simulink model "Project2"  (R2021a)
settings: Solver=VariableStepAuto  StartTime=0.0  StopTime=16  RelTol=1e-3
libraries: hdlBasic x209, dspsrcs4 x2, xbsIndex_r4 x1, hlsBasic x1
(part 1 of 2)
settings Model: Creator=caval  LastModifiedBy=user

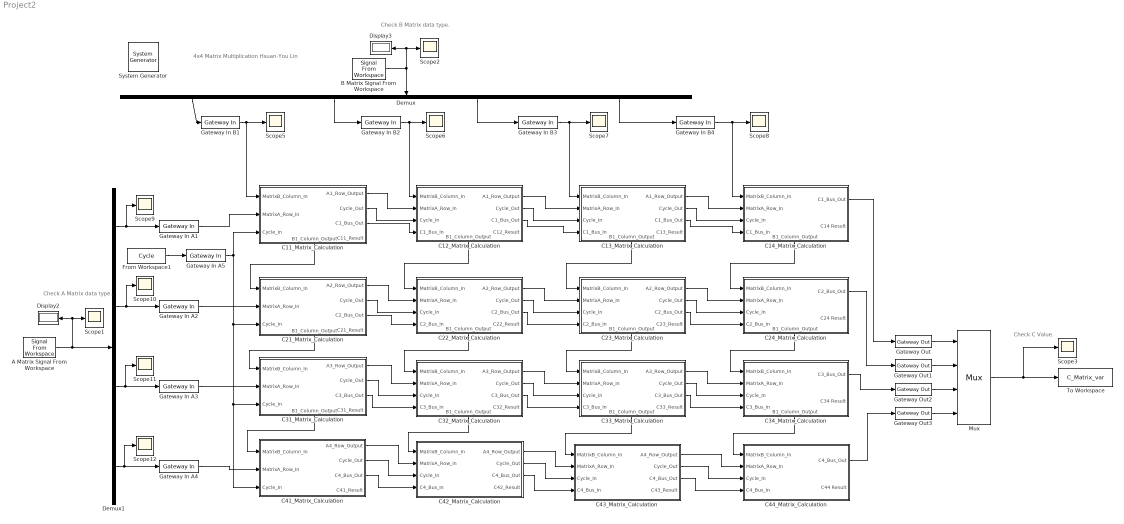
== system Project2 ==
  note: 4x4 Matrix Multiplication
      | Hsuan-You Lin
  note: Check A Matrix data type.
  note: Check B Matrix data type.
  note: Check C Value.
  " System Generator" : xbsIndex_r4/ System Generator  Tag=genX  xilinxfamily=zynq  part=xc7z020  speed=-1  package=clg484  synthesis_tool=Vivado  clock_wrapper=Clock Enables  directory=./netlist  proj_type=Vivado  Synth_file=Vivado Synthesis Defaults  Impl_file=Vivado Implementation Defaults  testbench=off  simulink_period=1  sysclk_period=7  dcm_input_clock_period=10  incr_netlist=off  trim_vbits=Everywhere in SubSystem  dbl_ovrd=According to Block Masks  core_generation=According to Block Masks  run_coregen=off  deprecated_control=off  eval_field=0  block_type=sysgen
  A Matrix Signal From Workspace : dspsrcs4/Signal From Workspace  X=A_Input  Ts=1  nsamps=1  OutputAfterFinalValue=Setting to zero  ignoreOrWarnInputAndFrameLengths=off  OutputFrames=off
  B Matrix Signal From Workspace : dspsrcs4/Signal From Workspace  X=B_Input  Ts=1  nsamps=1  OutputAfterFinalValue=Setting to zero  ignoreOrWarnInputAndFrameLengths=off  OutputFrames=off
  C11_Matrix_Calculation : Subsystem
      settings: PortSchema="{\"entries\":[{\"content\":{\"sides\":[{\"content\":{\"connectorIds\":[\"In1\",\"In2\",\"In3\"]},\"type\":\"ConnectorPlacement.EquallySpacedRectSide\",\"uuid\":\"74ab6ecd-cc08-4ee4-ac19-9cc8be9c6472\"},{\"content\":{\"connectorIds\":[\"Out1\",\"Out2\",\"Out3\",\"Out4\"],\"side\":\"RIGHT\"},\"type\":\"ConnectorPlacement.EquallySpacedRectSide\",\"uuid\":\"1cd07b35-dcc9-4612-a415-f960f8d5f61b\"},{\"content\":{\"connectorIds\":[],\"side\":\"TOP\"},\"type\":\"ConnectorPlacement.EquallySpacedRectSide\",\"uuid\":\"476a3fdc-a239-49e7-9d04-c8df306fd8f0\"},{\"content\":{\"connectorIds\":[\"Out5\"],\"side\":\"BOTTOM\"},\"type\":\"ConnectorPlacement.EquallySpacedRectSide\",\"uuid\":\"4811719c-b9ad-4f94-b919-bfccafa53e00\"}]},\"type\":\"ConnectorPlacement.EquallySpacedConnector\",\"uuid\":\"06e904f9-bca4-4dcb-a7b8-01e13ea2fc40\"}],\"packageUris\":[\"http://schema.mathworks.com/mf0/Connector/R2020b\"],\"version\":\"1.0\"}"
  C12_Matrix_Calculation : Subsystem
      settings: PortSchema="{\"entries\":[{\"content\":{\"sides\":[{\"content\":{\"connectorIds\":[\"In1\",\"In2\",\"In3\",\"In4\"]},\"type\":\"ConnectorPlacement.EquallySpacedRectSide\",\"uuid\":\"74ab6ecd-cc08-4ee4-ac19-9cc8be9c6472\"},{\"content\":{\"connectorIds\":[\"Out1\",\"Out2\",\"Out3\",\"Out4\"],\"side\":\"RIGHT\"},\"type\":\"ConnectorPlacement.EquallySpacedRectSide\",\"uuid\":\"1cd07b35-dcc9-4612-a415-f960f8d5f61b\"},{\"content\":{\"connectorIds\":[],\"side\":\"TOP\"},\"type\":\"ConnectorPlacement.EquallySpacedRectSide\",\"uuid\":\"476a3fdc-a239-49e7-9d04-c8df306fd8f0\"},{\"content\":{\"connectorIds\":[\"Out5\"],\"side\":\"BOTTOM\"},\"type\":\"ConnectorPlacement.EquallySpacedRectSide\",\"uuid\":\"4811719c-b9ad-4f94-b919-bfccafa53e00\"}]},\"type\":\"ConnectorPlacement.EquallySpacedConnector\",\"uuid\":\"06e904f9-bca4-4dcb-a7b8-01e13ea2fc40\"}],\"packageUris\":[\"http://schema.mathworks.com/mf0/Connector/R2020b\"],\"version\":\"1.0\"}"
  C13_Matrix_Calculation : Subsystem
      settings: PortSchema="{\"entries\":[{\"content\":{\"sides\":[{\"content\":{\"connectorIds\":[\"In1\",\"In2\",\"In3\",\"In4\"]},\"type\":\"ConnectorPlacement.EquallySpacedRectSide\",\"uuid\":\"74ab6ecd-cc08-4ee4-ac19-9cc8be9c6472\"},{\"content\":{\"connectorIds\":[\"Out1\",\"Out2\",\"Out3\",\"Out4\"],\"side\":\"RIGHT\"},\"type\":\"ConnectorPlacement.EquallySpacedRectSide\",\"uuid\":\"1cd07b35-dcc9-4612-a415-f960f8d5f61b\"},{\"content\":{\"connectorIds\":[],\"side\":\"TOP\"},\"type\":\"ConnectorPlacement.EquallySpacedRectSide\",\"uuid\":\"476a3fdc-a239-49e7-9d04-c8df306fd8f0\"},{\"content\":{\"connectorIds\":[\"Out5\"],\"side\":\"BOTTOM\"},\"type\":\"ConnectorPlacement.EquallySpacedRectSide\",\"uuid\":\"4811719c-b9ad-4f94-b919-bfccafa53e00\"}]},\"type\":\"ConnectorPlacement.EquallySpacedConnector\",\"uuid\":\"06e904f9-bca4-4dcb-a7b8-01e13ea2fc40\"}],\"packageUris\":[\"http://schema.mathworks.com/mf0/Connector/R2020b\"],\"version\":\"1.0\"}"
  C14_Matrix_Calculation : Subsystem
      settings: PortSchema="{\"entries\":[{\"content\":{\"sides\":[{\"content\":{\"connectorIds\":[\"In1\",\"In2\",\"In3\",\"In4\"]},\"type\":\"ConnectorPlacement.EquallySpacedRectSide\",\"uuid\":\"74ab6ecd-cc08-4ee4-ac19-9cc8be9c6472\"},{\"content\":{\"connectorIds\":[\"Out1\",\"Out2\"],\"side\":\"RIGHT\"},\"type\":\"ConnectorPlacement.EquallySpacedRectSide\",\"uuid\":\"1cd07b35-dcc9-4612-a415-f960f8d5f61b\"},{\"content\":{\"connectorIds\":[],\"side\":\"TOP\"},\"type\":\"ConnectorPlacement.EquallySpacedRectSide\",\"uuid\":\"476a3fdc-a239-49e7-9d04-c8df306fd8f0\"},{\"content\":{\"connectorIds\":[\"Out3\"],\"side\":\"BOTTOM\"},\"type\":\"ConnectorPlacement.EquallySpacedRectSide\",\"uuid\":\"4811719c-b9ad-4f94-b919-bfccafa53e00\"}]},\"type\":\"ConnectorPlacement.EquallySpacedConnector\",\"uuid\":\"06e904f9-bca4-4dcb-a7b8-01e13ea2fc40\"}],\"packageUris\":[\"http://schema.mathworks.com/mf0/Connector/R2020b\"],\"version\":\"1.0\"}"
  C21_Matrix_Calculation : Subsystem
      settings: PortSchema="{\"entries\":[{\"content\":{\"sides\":[{\"content\":{\"connectorIds\":[\"In1\",\"In2\",\"In3\"]},\"type\":\"ConnectorPlacement.EquallySpacedRectSide\",\"uuid\":\"74ab6ecd-cc08-4ee4-ac19-9cc8be9c6472\"},{\"content\":{\"connectorIds\":[\"Out1\",\"Out2\",\"Out3\",\"Out4\"],\"side\":\"RIGHT\"},\"type\":\"ConnectorPlacement.EquallySpacedRectSide\",\"uuid\":\"1cd07b35-dcc9-4612-a415-f960f8d5f61b\"},{\"content\":{\"connectorIds\":[],\"side\":\"TOP\"},\"type\":\"ConnectorPlacement.EquallySpacedRectSide\",\"uuid\":\"476a3fdc-a239-49e7-9d04-c8df306fd8f0\"},{\"content\":{\"connectorIds\":[\"Out5\"],\"side\":\"BOTTOM\"},\"type\":\"ConnectorPlacement.EquallySpacedRectSide\",\"uuid\":\"4811719c-b9ad-4f94-b919-bfccafa53e00\"}]},\"type\":\"ConnectorPlacement.EquallySpacedConnector\",\"uuid\":\"06e904f9-bca4-4dcb-a7b8-01e13ea2fc40\"}],\"packageUris\":[\"http://schema.mathworks.com/mf0/Connector/R2020b\"],\"version\":\"1.0\"}"
  C22_Matrix_Calculation : Subsystem
      settings: PortSchema="{\"entries\":[{\"content\":{\"sides\":[{\"content\":{\"connectorIds\":[\"In1\",\"In2\",\"In3\",\"In4\"]},\"type\":\"ConnectorPlacement.EquallySpacedRectSide\",\"uuid\":\"74ab6ecd-cc08-4ee4-ac19-9cc8be9c6472\"},{\"content\":{\"connectorIds\":[\"Out1\",\"Out2\",\"Out3\",\"Out4\"],\"side\":\"RIGHT\"},\"type\":\"ConnectorPlacement.EquallySpacedRectSide\",\"uuid\":\"1cd07b35-dcc9-4612-a415-f960f8d5f61b\"},{\"content\":{\"connectorIds\":[],\"side\":\"TOP\"},\"type\":\"ConnectorPlacement.EquallySpacedRectSide\",\"uuid\":\"476a3fdc-a239-49e7-9d04-c8df306fd8f0\"},{\"content\":{\"connectorIds\":[\"Out5\"],\"side\":\"BOTTOM\"},\"type\":\"ConnectorPlacement.EquallySpacedRectSide\",\"uuid\":\"4811719c-b9ad-4f94-b919-bfccafa53e00\"}]},\"type\":\"ConnectorPlacement.EquallySpacedConnector\",\"uuid\":\"06e904f9-bca4-4dcb-a7b8-01e13ea2fc40\"}],\"packageUris\":[\"http://schema.mathworks.com/mf0/Connector/R2020b\"],\"version\":\"1.0\"}"
  C23_Matrix_Calculation : Subsystem
      settings: PortSchema="{\"entries\":[{\"content\":{\"sides\":[{\"content\":{\"connectorIds\":[\"In1\",\"In2\",\"In3\",\"In4\"]},\"type\":\"ConnectorPlacement.EquallySpacedRectSide\",\"uuid\":\"74ab6ecd-cc08-4ee4-ac19-9cc8be9c6472\"},{\"content\":{\"connectorIds\":[\"Out1\",\"Out2\",\"Out3\",\"Out4\"],\"side\":\"RIGHT\"},\"type\":\"ConnectorPlacement.EquallySpacedRectSide\",\"uuid\":\"1cd07b35-dcc9-4612-a415-f960f8d5f61b\"},{\"content\":{\"connectorIds\":[],\"side\":\"TOP\"},\"type\":\"ConnectorPlacement.EquallySpacedRectSide\",\"uuid\":\"476a3fdc-a239-49e7-9d04-c8df306fd8f0\"},{\"content\":{\"connectorIds\":[\"Out5\"],\"side\":\"BOTTOM\"},\"type\":\"ConnectorPlacement.EquallySpacedRectSide\",\"uuid\":\"4811719c-b9ad-4f94-b919-bfccafa53e00\"}]},\"type\":\"ConnectorPlacement.EquallySpacedConnector\",\"uuid\":\"06e904f9-bca4-4dcb-a7b8-01e13ea2fc40\"}],\"packageUris\":[\"http://schema.mathworks.com/mf0/Connector/R2020b\"],\"version\":\"1.0\"}"
  C24_Matrix_Calculation : Subsystem
      settings: PortSchema="{\"entries\":[{\"content\":{\"sides\":[{\"content\":{\"connectorIds\":[\"In1\",\"In2\",\"In3\",\"In4\"]},\"type\":\"ConnectorPlacement.EquallySpacedRectSide\",\"uuid\":\"74ab6ecd-cc08-4ee4-ac19-9cc8be9c6472\"},{\"content\":{\"connectorIds\":[\"Out1\",\"Out2\"],\"side\":\"RIGHT\"},\"type\":\"ConnectorPlacement.EquallySpacedRectSide\",\"uuid\":\"1cd07b35-dcc9-4612-a415-f960f8d5f61b\"},{\"content\":{\"connectorIds\":[],\"side\":\"TOP\"},\"type\":\"ConnectorPlacement.EquallySpacedRectSide\",\"uuid\":\"476a3fdc-a239-49e7-9d04-c8df306fd8f0\"},{\"content\":{\"connectorIds\":[\"Out3\"],\"side\":\"BOTTOM\"},\"type\":\"ConnectorPlacement.EquallySpacedRectSide\",\"uuid\":\"4811719c-b9ad-4f94-b919-bfccafa53e00\"}]},\"type\":\"ConnectorPlacement.EquallySpacedConnector\",\"uuid\":\"06e904f9-bca4-4dcb-a7b8-01e13ea2fc40\"}],\"packageUris\":[\"http://schema.mathworks.com/mf0/Connector/R2020b\"],\"version\":\"1.0\"}"
  C31_Matrix_Calculation : Subsystem
      settings: PortSchema="{\"entries\":[{\"content\":{\"sides\":[{\"content\":{\"connectorIds\":[\"In1\",\"In2\",\"In3\"]},\"type\":\"ConnectorPlacement.EquallySpacedRectSide\",\"uuid\":\"74ab6ecd-cc08-4ee4-ac19-9cc8be9c6472\"},{\"content\":{\"connectorIds\":[\"Out1\",\"Out2\",\"Out3\",\"Out4\"],\"side\":\"RIGHT\"},\"type\":\"ConnectorPlacement.EquallySpacedRectSide\",\"uuid\":\"1cd07b35-dcc9-4612-a415-f960f8d5f61b\"},{\"content\":{\"connectorIds\":[],\"side\":\"TOP\"},\"type\":\"ConnectorPlacement.EquallySpacedRectSide\",\"uuid\":\"476a3fdc-a239-49e7-9d04-c8df306fd8f0\"},{\"content\":{\"connectorIds\":[\"Out5\"],\"side\":\"BOTTOM\"},\"type\":\"ConnectorPlacement.EquallySpacedRectSide\",\"uuid\":\"4811719c-b9ad-4f94-b919-bfccafa53e00\"}]},\"type\":\"ConnectorPlacement.EquallySpacedConnector\",\"uuid\":\"06e904f9-bca4-4dcb-a7b8-01e13ea2fc40\"}],\"packageUris\":[\"http://schema.mathworks.com/mf0/Connector/R2020b\"],\"version\":\"1.0\"}"
  C32_Matrix_Calculation : Subsystem
      settings: PortSchema="{\"entries\":[{\"content\":{\"sides\":[{\"content\":{\"connectorIds\":[\"In1\",\"In2\",\"In3\",\"In4\"]},\"type\":\"ConnectorPlacement.EquallySpacedRectSide\",\"uuid\":\"74ab6ecd-cc08-4ee4-ac19-9cc8be9c6472\"},{\"content\":{\"connectorIds\":[\"Out1\",\"Out2\",\"Out3\",\"Out4\"],\"side\":\"RIGHT\"},\"type\":\"ConnectorPlacement.EquallySpacedRectSide\",\"uuid\":\"1cd07b35-dcc9-4612-a415-f960f8d5f61b\"},{\"content\":{\"connectorIds\":[],\"side\":\"TOP\"},\"type\":\"ConnectorPlacement.EquallySpacedRectSide\",\"uuid\":\"476a3fdc-a239-49e7-9d04-c8df306fd8f0\"},{\"content\":{\"connectorIds\":[\"Out5\"],\"side\":\"BOTTOM\"},\"type\":\"ConnectorPlacement.EquallySpacedRectSide\",\"uuid\":\"4811719c-b9ad-4f94-b919-bfccafa53e00\"}]},\"type\":\"ConnectorPlacement.EquallySpacedConnector\",\"uuid\":\"06e904f9-bca4-4dcb-a7b8-01e13ea2fc40\"}],\"packageUris\":[\"http://schema.mathworks.com/mf0/Connector/R2020b\"],\"version\":\"1.0\"}"
  C33_Matrix_Calculation : Subsystem
      settings: PortSchema="{\"entries\":[{\"content\":{\"sides\":[{\"content\":{\"connectorIds\":[\"In1\",\"In2\",\"In3\",\"In4\"]},\"type\":\"ConnectorPlacement.EquallySpacedRectSide\",\"uuid\":\"74ab6ecd-cc08-4ee4-ac19-9cc8be9c6472\"},{\"content\":{\"connectorIds\":[\"Out1\",\"Out2\",\"Out3\",\"Out4\"],\"side\":\"RIGHT\"},\"type\":\"ConnectorPlacement.EquallySpacedRectSide\",\"uuid\":\"1cd07b35-dcc9-4612-a415-f960f8d5f61b\"},{\"content\":{\"connectorIds\":[],\"side\":\"TOP\"},\"type\":\"ConnectorPlacement.EquallySpacedRectSide\",\"uuid\":\"476a3fdc-a239-49e7-9d04-c8df306fd8f0\"},{\"content\":{\"connectorIds\":[\"Out5\"],\"side\":\"BOTTOM\"},\"type\":\"ConnectorPlacement.EquallySpacedRectSide\",\"uuid\":\"4811719c-b9ad-4f94-b919-bfccafa53e00\"}]},\"type\":\"ConnectorPlacement.EquallySpacedConnector\",\"uuid\":\"06e904f9-bca4-4dcb-a7b8-01e13ea2fc40\"}],\"packageUris\":[\"http://schema.mathworks.com/mf0/Connector/R2020b\"],\"version\":\"1.0\"}"
  C34_Matrix_Calculation : Subsystem
      settings: PortSchema="{\"entries\":[{\"content\":{\"sides\":[{\"content\":{\"connectorIds\":[\"In1\",\"In2\",\"In3\",\"In4\"]},\"type\":\"ConnectorPlacement.EquallySpacedRectSide\",\"uuid\":\"74ab6ecd-cc08-4ee4-ac19-9cc8be9c6472\"},{\"content\":{\"connectorIds\":[\"Out1\",\"Out2\"],\"side\":\"RIGHT\"},\"type\":\"ConnectorPlacement.EquallySpacedRectSide\",\"uuid\":\"1cd07b35-dcc9-4612-a415-f960f8d5f61b\"},{\"content\":{\"connectorIds\":[],\"side\":\"TOP\"},\"type\":\"ConnectorPlacement.EquallySpacedRectSide\",\"uuid\":\"476a3fdc-a239-49e7-9d04-c8df306fd8f0\"},{\"content\":{\"connectorIds\":[\"Out3\"],\"side\":\"BOTTOM\"},\"type\":\"ConnectorPlacement.EquallySpacedRectSide\",\"uuid\":\"4811719c-b9ad-4f94-b919-bfccafa53e00\"}]},\"type\":\"ConnectorPlacement.EquallySpacedConnector\",\"uuid\":\"06e904f9-bca4-4dcb-a7b8-01e13ea2fc40\"}],\"packageUris\":[\"http://schema.mathworks.com/mf0/Connector/R2020b\"],\"version\":\"1.0\"}"
  C41_Matrix_Calculation : Subsystem
  C42_Matrix_Calculation : Subsystem
  C43_Matrix_Calculation : Subsystem
  C44_Matrix_Calculation : Subsystem
  Demux : Demux
  Demux1 : Demux
  Display2 : Display
  Display3 : Display
  From Workspace1 : FromWorkspace  VariableName=Cycle
  Gateway In A{1..5} (5 alike) : hdlBasic/Gateway In  gui_display_data_type=Fixed-point  arith_type=Signed (2's comp)  n_bits=16  bin_pt=0  preci_type=Single  exp_width=8  frac_width=24  rows=1  columns=1  quantization="Round  (unbiased: +/- Inf)"  overflow=Saturate  period=1  UseAsADC=off  ADCChannel='1'  interface=None  automatic_assignment=on  address_offset=hex2dec('00')  intf_name=''  intf_description=''  default_value=0  timing_constraint=None  locs_specified=off  LOCs={}  io_standard={}  inherit_from_input=off  hdl_port=on  XmcBlockStatus=1  maskContainerNames=group4  block_type=gatewayin  block_config=sysgen:gateway_in_config  block_width_w=590  block_height_w=620  block_width=640  block_height=850
  Gateway In B{1..4} (4 alike) : hdlBasic/Gateway In  gui_display_data_type=Fixed-point  arith_type=Signed (2's comp)  n_bits=16  bin_pt=0  preci_type=Single  exp_width=8  frac_width=24  rows=1  columns=1  quantization="Round  (unbiased: +/- Inf)"  overflow=Saturate  period=1  UseAsADC=off  ADCChannel='1'  interface=None  automatic_assignment=on  address_offset=hex2dec('00')  intf_name=''  intf_description=''  default_value=0  timing_constraint=None  locs_specified=off  LOCs={}  io_standard={}  inherit_from_input=off  hdl_port=on  XmcBlockStatus=1  maskContainerNames=group4  block_type=gatewayin  block_config=sysgen:gateway_in_config  block_width_w=590  block_height_w=620  block_width=640  block_height=850
  Gateway Out{,1..3} (4 alike) : hdlBasic/Gateway Out  inherit_from_input=off  hdl_port=on  rows=1  columns=1  UseAsDAC=off  DACChannel='1'  interface=None  automatic_assignment=on  address_offset=hex2dec('00')  intf_name=''  intf_description=''  timing_constraint=None  locs_specified=off  LOCs={}  io_standard={}  XmcBlockStatus=1  maskContainerNames=group4  block_type=gatewayout  block_config=sysgen:gateway_out_config  block_width_w=590  block_height_w=620  block_width=620  block_height=750
  Mux : hlsBasic/Mux  NumInputs=4
  Scope{1..3,5..12} (11 alike) : Scope
  To Workspace : ToWorkspace  VariableName=C_Matrix_var  SaveFormat=Timeseries  SampleTime=-1
  wires:
  Gateway In B1/1 -> C11_Matrix_Calculation/1(MatrixB_Column_In), Scope5/1
  Gateway In A1/1 -> C11_Matrix_Calculation/2(MatrixA_Row_In)
  C11_Matrix_Calculation/1(A1_Row_Output) -> C12_Matrix_Calculation/2(MatrixA_Row_In)
  C12_Matrix_Calculation/1(A1_Row_Output) -> C13_Matrix_Calculation/2(MatrixA_Row_In)
  C13_Matrix_Calculation/1(A1_Row_Output) -> C14_Matrix_Calculation/2(MatrixA_Row_In)
  C11_Matrix_Calculation/5(B1_Column_Output) -> C21_Matrix_Calculation/1(MatrixB_Column_In)
  C12_Matrix_Calculation/5(B1_Column_Output) -> C22_Matrix_Calculation/1(MatrixB_Column_In)
  C14_Matrix_Calculation/3(B1_Column_Output) -> C24_Matrix_Calculation/1(MatrixB_Column_In)
  C21_Matrix_Calculation/5(B1_Column_Output) -> C31_Matrix_Calculation/1(MatrixB_Column_In)
  B Matrix Signal From Workspace/1 -> Scope2/1, Display3/1, Demux/1
  Demux1/1 -> Scope9/1, Gateway In A1/1
  Demux1/2 -> Gateway In A2/1, Scope10/1
  Demux1/3 -> Gateway In A3/1, Scope11/1
  Demux1/4 -> Scope12/1, Gateway In A4/1
  A Matrix Signal From Workspace/1 -> Scope1/1, Display2/1, Demux1/1
  Demux/1 -> Gateway In B1/1
  Demux/2 -> Gateway In B2/1
  Demux/3 -> Gateway In B3/1
  Demux/4 -> Gateway In B4/1
  Gateway In A3/1 -> C31_Matrix_Calculation/2(MatrixA_Row_In)
  Gateway In A4/1 -> C41_Matrix_Calculation/2(MatrixA_Row_In)
  Gateway In B2/1 -> C12_Matrix_Calculation/1(MatrixB_Column_In), Scope6/1
  Gateway In B3/1 -> C13_Matrix_Calculation/1(MatrixB_Column_In), Scope7/1
  Gateway In B4/1 -> C14_Matrix_Calculation/1(MatrixB_Column_In), Scope8/1
  Gateway Out/1 -> Mux/1
  Gateway Out1/1 -> Mux/2
  Gateway Out2/1 -> Mux/3
  Gateway Out3/1 -> Mux/4
  Mux/1 -> To Workspace/1, Scope3/1
  From Workspace1/1 -> Gateway In A5/1
  Gateway In A5/1 -> C11_Matrix_Calculation/3(Cycle_In), C41_Matrix_Calculation/3(Cycle_In), C31_Matrix_Calculation/3(Cycle_In), C21_Matrix_Calculation/3(Cycle_In)
  C11_Matrix_Calculation/3(C1_Bus_Out) -> C12_Matrix_Calculation/4(C1_Bus_In)
  C11_Matrix_Calculation/2(Cycle_Out) -> C12_Matrix_Calculation/3(Cycle_In)
  C12_Matrix_Calculation/2(Cycle_Out) -> C13_Matrix_Calculation/3(Cycle_In)
  C12_Matrix_Calculation/3(C1_Bus_Out) -> C13_Matrix_Calculation/4(C1_Bus_In)
  C13_Matrix_Calculation/2(Cycle_Out) -> C14_Matrix_Calculation/3(Cycle_In)
  C13_Matrix_Calculation/3(C1_Bus_Out) -> C14_Matrix_Calculation/4(C1_Bus_In)
  C14_Matrix_Calculation/1(C1_Bus_Out) -> Gateway Out/1
  Gateway In A2/1 -> C21_Matrix_Calculation/2(MatrixA_Row_In)
  C31_Matrix_Calculation/5(B1_Column_Output) -> C41_Matrix_Calculation/1(MatrixB_Column_In)
  C21_Matrix_Calculation/1(A2_Row_Output) -> C22_Matrix_Calculation/2(MatrixA_Row_In)
  C21_Matrix_Calculation/2(Cycle_Out) -> C22_Matrix_Calculation/3(Cycle_In)
  C21_Matrix_Calculation/3(C2_Bus_Out) -> C22_Matrix_Calculation/4(C2_Bus_In)
  C31_Matrix_Calculation/1(A3_Row_Output) -> C32_Matrix_Calculation/2(MatrixA_Row_In)
  C22_Matrix_Calculation/5(B1_Column_Output) -> C32_Matrix_Calculation/1(MatrixB_Column_In)
  C31_Matrix_Calculation/2(Cycle_Out) -> C32_Matrix_Calculation/3(Cycle_In)
  C31_Matrix_Calculation/3(C3_Bus_Out) -> C32_Matrix_Calculation/4(C3_Bus_In)
  C32_Matrix_Calculation/5(B1_Column_Output) -> C42_Matrix_Calculation/1(MatrixB_Column_In)
  C41_Matrix_Calculation/1(A4_Row_Output) -> C42_Matrix_Calculation/2(MatrixA_Row_In)
  C41_Matrix_Calculation/2(Cycle_Out) -> C42_Matrix_Calculation/3(Cycle_In)
  C41_Matrix_Calculation/3(C4_Bus_Out) -> C42_Matrix_Calculation/4(C4_Bus_In)
  C13_Matrix_Calculation/5(B1_Column_Output) -> C23_Matrix_Calculation/1(MatrixB_Column_In)
  C22_Matrix_Calculation/1(A2_Row_Output) -> C23_Matrix_Calculation/2(MatrixA_Row_In)
  C22_Matrix_Calculation/2(Cycle_Out) -> C23_Matrix_Calculation/3(Cycle_In)
  C22_Matrix_Calculation/3(C2_Bus_Out) -> C23_Matrix_Calculation/4(C2_Bus_In)
  C23_Matrix_Calculation/5(B1_Column_Output) -> C33_Matrix_Calculation/1(MatrixB_Column_In)
  C32_Matrix_Calculation/1(A3_Row_Output) -> C33_Matrix_Calculation/2(MatrixA_Row_In)
  C32_Matrix_Calculation/2(Cycle_Out) -> C33_Matrix_Calculation/3(Cycle_In)
  C32_Matrix_Calculation/3(C3_Bus_Out) -> C33_Matrix_Calculation/4(C3_Bus_In)
  C33_Matrix_Calculation/5(B1_Column_Output) -> C43_Matrix_Calculation/1(MatrixB_Column_In)
  C42_Matrix_Calculation/1(A4_Row_Output) -> C43_Matrix_Calculation/2(MatrixA_Row_In)
  C42_Matrix_Calculation/2(Cycle_Out) -> C43_Matrix_Calculation/3(Cycle_In)
  C42_Matrix_Calculation/3(C4_Bus_Out) -> C43_Matrix_Calculation/4(C4_Bus_In)
  C23_Matrix_Calculation/1(A2_Row_Output) -> C24_Matrix_Calculation/2(MatrixA_Row_In)
  C23_Matrix_Calculation/2(Cycle_Out) -> C24_Matrix_Calculation/3(Cycle_In)
  C23_Matrix_Calculation/3(C2_Bus_Out) -> C24_Matrix_Calculation/4(C2_Bus_In)
  C24_Matrix_Calculation/1(C2_Bus_Out) -> Gateway Out1/1
  C24_Matrix_Calculation/3(B1_Column_Output) -> C34_Matrix_Calculation/1(MatrixB_Column_In)
  C33_Matrix_Calculation/1(A3_Row_Output) -> C34_Matrix_Calculation/2(MatrixA_Row_In)
  C33_Matrix_Calculation/2(Cycle_Out) -> C34_Matrix_Calculation/3(Cycle_In)
  C33_Matrix_Calculation/3(C3_Bus_Out) -> C34_Matrix_Calculation/4(C3_Bus_In)
  C34_Matrix_Calculation/3(B1_Column_Output) -> C44_Matrix_Calculation/1(MatrixB_Column_In)
  C43_Matrix_Calculation/1(A4_Row_Output) -> C44_Matrix_Calculation/2(MatrixA_Row_In)
  C43_Matrix_Calculation/2(Cycle_Out) -> C44_Matrix_Calculation/3(Cycle_In)
  C43_Matrix_Calculation/3(C4_Bus_Out) -> C44_Matrix_Calculation/4(C4_Bus_In)
  C44_Matrix_Calculation/1(C4_Bus_Out) -> Gateway Out3/1
  C34_Matrix_Calculation/1(C3_Bus_Out) -> Gateway Out2/1

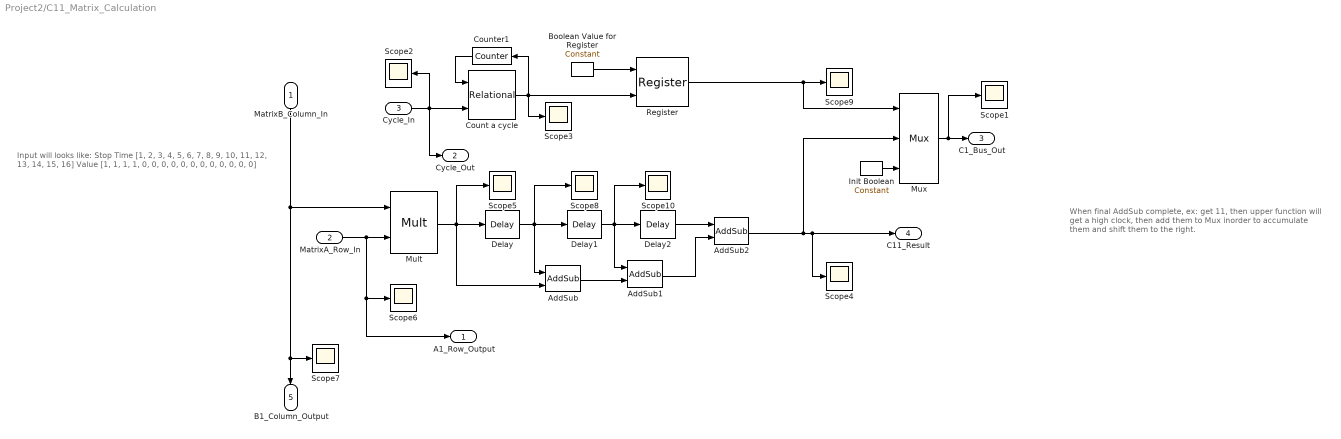
== system Project2/C11_Matrix_Calculation ==
  note: Input will looks like:
      | Stop Time [1, 2, 3, 4, 5, 6, 7, 8, 9, 10, 11, 12, 13, 14, 15, 16]
      | Value [1, 1, 1, 1, 0, 0, 0, 0, 0, 0, 0, 0, 0, 0, 0, 0]
  note: When final AddSub complete, ex: get 11, then upper function will get a high clock, then add them to Mux inorder to accumulate them and shift them to the right.
  MatrixB_Column_In : Inport
  MatrixA_Row_In : Inport  Port=2
  Cycle_In : Inport  Port=3
  AddSub : hdlBasic/AddSub  mode=Addition  use_carryin=off  use_carryout=off  en=off  latency=0  precision=Full  arith_type=Unsigned  n_bits=16  bin_pt=14  quantization=Truncate  overflow=Wrap  use_behavioral_HDL=off  hw_selection=Fabric  pipelined=off  XmcBlockStatus=1  maskContainerNames=tabcontainer1  block_type=addsub  block_config=sysgen:Addsub_config
  AddSub1 : hdlBasic/AddSub  mode=Addition  use_carryin=off  use_carryout=off  en=off  latency=0  precision=Full  arith_type=Unsigned  n_bits=16  bin_pt=14  quantization=Truncate  overflow=Wrap  use_behavioral_HDL=off  hw_selection=Fabric  pipelined=off  XmcBlockStatus=1  maskContainerNames=tabcontainer1  block_type=addsub  block_config=sysgen:Addsub_config
  AddSub2 : hdlBasic/AddSub  mode=Addition  use_carryin=off  use_carryout=off  en=off  latency=0  precision=Full  arith_type=Unsigned  n_bits=16  bin_pt=14  quantization=Truncate  overflow=Wrap  use_behavioral_HDL=off  hw_selection=Fabric  pipelined=off  XmcBlockStatus=1  maskContainerNames=tabcontainer1  block_type=addsub  block_config=sysgen:Addsub_config
  Boolean Value for Register : hdlBasic/Constant  const=1.0  gui_display_data_type=Boolean  arith_type=Boolean  n_bits=16  bin_pt=14  preci_type=Single  exp_width=8  frac_width=24  explicit_period=off  period=1  XmcBlockStatus=1  maskContainerNames=tabcontainer1  block_type=constant  block_config=sysgen:Constant_config
  Count a cycle : hdlBasic/Relational  mode=a=b  op_type=Bool  en=off  latency=1  XmcBlockStatus=1  maskContainerNames=tabcontainer1  block_type=relational  block_config=sysgen:Relational_config
  Counter1 : hdlBasic/Counter  cnt_type=Free running  cnt_to=8  operation=Up  start_count=0  cnt_by_val=1  arith_type=Unsigned  n_bits=6  bin_pt=0  load_pin=off  rst=on  en=off  explicit_period=Explicit  period=1  use_behavioral_HDL=off  implementation=Fabric  XmcBlockStatus=1  maskContainerNames=group1  block_type=counter  block_config=sysgen:Counter_config
  Delay : hdlBasic/Delay  rst=off  en=off  latency=1  reg_retiming=off  XmcBlockStatus=1  maskContainerNames=group1  block_type=delay  block_config=sysgen:Delay_config
  Delay1 : hdlBasic/Delay  rst=off  en=off  latency=1  reg_retiming=off  XmcBlockStatus=1  maskContainerNames=group1  block_type=delay  block_config=sysgen:Delay_config
  Delay2 : hdlBasic/Delay  rst=off  en=off  latency=1  reg_retiming=off  XmcBlockStatus=1  maskContainerNames=group1  block_type=delay  block_config=sysgen:Delay_config
  Init Boolean : hdlBasic/Constant  const=0  gui_display_data_type=Fixed-point  arith_type=Signed (2's comp)  n_bits=16  bin_pt=14  preci_type=Single  exp_width=8  frac_width=24  explicit_period=off  period=1  XmcBlockStatus=1  maskContainerNames=tabcontainer1  block_type=constant  block_config=sysgen:Constant_config
  Mult : hdlBasic/Mult  precision=Full  arith_type="Signed  (2's comp)"  n_bits=16  bin_pt=14  quantization=Truncate  overflow=Wrap  en=off  latency=3  use_behavioral_HDL=off  opt=Speed  use_embedded=on  optimum_pipeline=off  pipeline=on  use_rpm=on  placement_style=Triangular  XmcBlockStatus=1  maskContainerNames=group1  block_type=mult  block_config=sysgen:Mult_config
  Mux : hdlBasic/Mux  inputs=2  en=off  latency=1  precision=Full  arith_type=Unsigned  n_bits=16  bin_pt=14  quantization=Truncate  overflow=Wrap  XmcBlockStatus=1  maskContainerNames=tabcontainer1  block_type=mux  block_config=sysgen:Mux_config
  Register : hdlBasic/Register  init=0  rst=on  en=off  XmcBlockStatus=1  maskContainerNames=tabcontainer1  block_type=register  block_config=sysgen:Register_config
  Scope{1..10} (10 alike) : Scope
  A1_Row_Output : Outport
  Cycle_Out : Outport  Port=2
  C1_Bus_Out : Outport  Port=3
  C11_Result : Outport  Port=4
  B1_Column_Output : Outport  Port=5
  wires:
  Mult/1 -> Scope5/1, Delay/1, AddSub/2
  AddSub/1 -> AddSub1/2
  Delay/1 -> Scope8/1, AddSub/1, Delay1/1
  Delay1/1 -> Scope10/1, Delay2/1, AddSub1/1
  AddSub1/1 -> AddSub2/2
  Delay2/1 -> AddSub2/1
  AddSub2/1 -> Scope4/1, C11_Result/1, Mux/2
  MatrixB_Column_In/1 -> Scope7/1, B1_Column_Output/1, Mult/1
  MatrixA_Row_In/1 -> Scope6/1, A1_Row_Output/1, Mult/2
  Counter1/1 -> Count a cycle/1
  Count a cycle/1 -> Register/2, Counter1/1, Scope3/1
  Boolean Value for Register/1 -> Register/1
  Register/1 -> Mux/1, Scope9/1
  Cycle_In/1 -> Cycle_Out/1, Count a cycle/2, Scope2/1
  Init Boolean/1 -> Mux/3
  Mux/1 -> Scope1/1, C1_Bus_Out/1

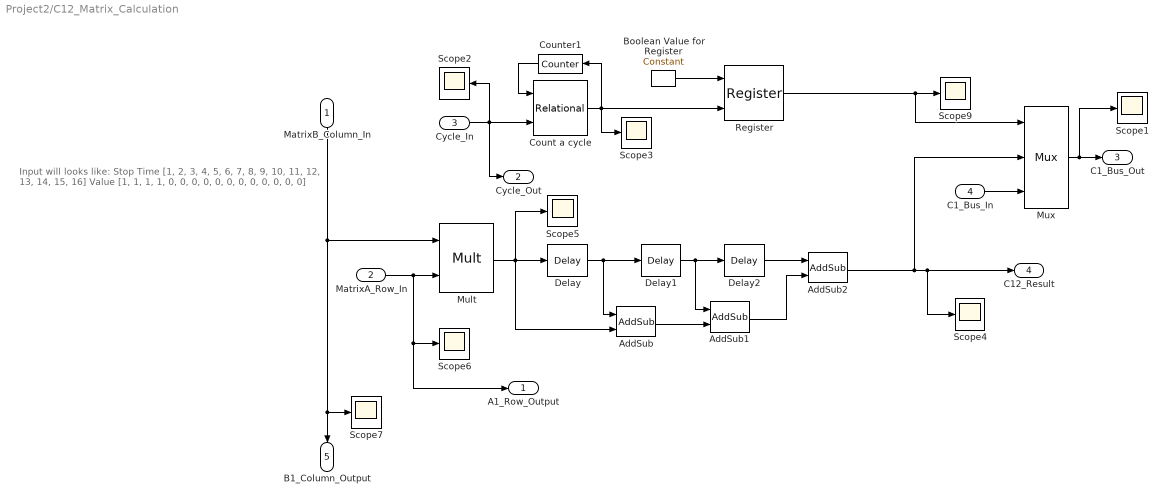
== system Project2/C12_Matrix_Calculation ==
  note: Input will looks like:
      | Stop Time [1, 2, 3, 4, 5, 6, 7, 8, 9, 10, 11, 12, 13, 14, 15, 16]
      | Value [1, 1, 1, 1, 0, 0, 0, 0, 0, 0, 0, 0, 0, 0, 0, 0]
  MatrixB_Column_In : Inport
  MatrixA_Row_In : Inport  Port=2
  Cycle_In : Inport  Port=3
  C1_Bus_In : Inport  Port=4
  AddSub : hdlBasic/AddSub  mode=Addition  use_carryin=off  use_carryout=off  en=off  latency=0  precision=Full  arith_type=Unsigned  n_bits=16  bin_pt=14  quantization=Truncate  overflow=Wrap  use_behavioral_HDL=off  hw_selection=Fabric  pipelined=off  XmcBlockStatus=1  maskContainerNames=tabcontainer1  block_type=addsub  block_config=sysgen:Addsub_config
  AddSub1 : hdlBasic/AddSub  mode=Addition  use_carryin=off  use_carryout=off  en=off  latency=0  precision=Full  arith_type=Unsigned  n_bits=16  bin_pt=14  quantization=Truncate  overflow=Wrap  use_behavioral_HDL=off  hw_selection=Fabric  pipelined=off  XmcBlockStatus=1  maskContainerNames=tabcontainer1  block_type=addsub  block_config=sysgen:Addsub_config
  AddSub2 : hdlBasic/AddSub  mode=Addition  use_carryin=off  use_carryout=off  en=off  latency=0  precision=Full  arith_type=Unsigned  n_bits=16  bin_pt=14  quantization=Truncate  overflow=Wrap  use_behavioral_HDL=off  hw_selection=Fabric  pipelined=off  XmcBlockStatus=1  maskContainerNames=tabcontainer1  block_type=addsub  block_config=sysgen:Addsub_config
  Boolean Value for Register : hdlBasic/Constant  const=1.0  gui_display_data_type=Boolean  arith_type=Boolean  n_bits=16  bin_pt=14  preci_type=Single  exp_width=8  frac_width=24  explicit_period=off  period=1  XmcBlockStatus=1  maskContainerNames=tabcontainer1  block_type=constant  block_config=sysgen:Constant_config
  Count a cycle : hdlBasic/Relational  mode=a=b  op_type=Bool  en=off  latency=1  XmcBlockStatus=1  maskContainerNames=tabcontainer1  block_type=relational  block_config=sysgen:Relational_config
  Counter1 : hdlBasic/Counter  cnt_type=Free running  cnt_to=8  operation=Up  start_count=0  cnt_by_val=1  arith_type=Unsigned  n_bits=6  bin_pt=0  load_pin=off  rst=on  en=off  explicit_period=Explicit  period=1  use_behavioral_HDL=off  implementation=Fabric  XmcBlockStatus=1  maskContainerNames=group1  block_type=counter  block_config=sysgen:Counter_config
  Delay : hdlBasic/Delay  rst=off  en=off  latency=1  reg_retiming=off  XmcBlockStatus=1  maskContainerNames=group1  block_type=delay  block_config=sysgen:Delay_config
  Delay1 : hdlBasic/Delay  rst=off  en=off  latency=1  reg_retiming=off  XmcBlockStatus=1  maskContainerNames=group1  block_type=delay  block_config=sysgen:Delay_config
  Delay2 : hdlBasic/Delay  rst=off  en=off  latency=1  reg_retiming=off  XmcBlockStatus=1  maskContainerNames=group1  block_type=delay  block_config=sysgen:Delay_config
  Mult : hdlBasic/Mult  precision=Full  arith_type="Signed  (2's comp)"  n_bits=16  bin_pt=14  quantization=Truncate  overflow=Wrap  en=off  latency=3  use_behavioral_HDL=off  opt=Speed  use_embedded=on  optimum_pipeline=off  pipeline=on  use_rpm=on  placement_style=Triangular  XmcBlockStatus=1  maskContainerNames=group1  block_type=mult  block_config=sysgen:Mult_config
  Mux : hdlBasic/Mux  inputs=2  en=off  latency=1  precision=Full  arith_type=Unsigned  n_bits=16  bin_pt=14  quantization=Truncate  overflow=Wrap  XmcBlockStatus=1  maskContainerNames=tabcontainer1  block_type=mux  block_config=sysgen:Mux_config
  Register : hdlBasic/Register  init=0  rst=on  en=off  XmcBlockStatus=1  maskContainerNames=tabcontainer1  block_type=register  block_config=sysgen:Register_config
  Scope{1..7,9} (8 alike) : Scope
  A1_Row_Output : Outport
  Cycle_Out : Outport  Port=2
  C1_Bus_Out : Outport  Port=3
  C12_Result : Outport  Port=4
  B1_Column_Output : Outport  Port=5
  wires:
  MatrixA_Row_In/1 -> Scope6/1, A1_Row_Output/1, Mult/2
  AddSub/1 -> AddSub1/2
  AddSub1/1 -> AddSub2/2
  Delay2/1 -> AddSub2/1
  Mult/1 -> Scope5/1, Delay/1, AddSub/2
  Delay1/1 -> Delay2/1, AddSub1/1
  Delay/1 -> AddSub/1, Delay1/1
  C1_Bus_In/1 -> Mux/3
  Mux/1 -> Scope1/1, C1_Bus_Out/1
  Register/1 -> Mux/1, Scope9/1
  Boolean Value for Register/1 -> Register/1
  Count a cycle/1 -> Register/2, Counter1/1, Scope3/1
  Counter1/1 -> Count a cycle/1
  AddSub2/1 -> Mux/2, Scope4/1, C12_Result/1
  MatrixB_Column_In/1 -> Mult/1, Scope7/1, B1_Column_Output/1
  Cycle_In/1 -> Cycle_Out/1, Count a cycle/2, Scope2/1

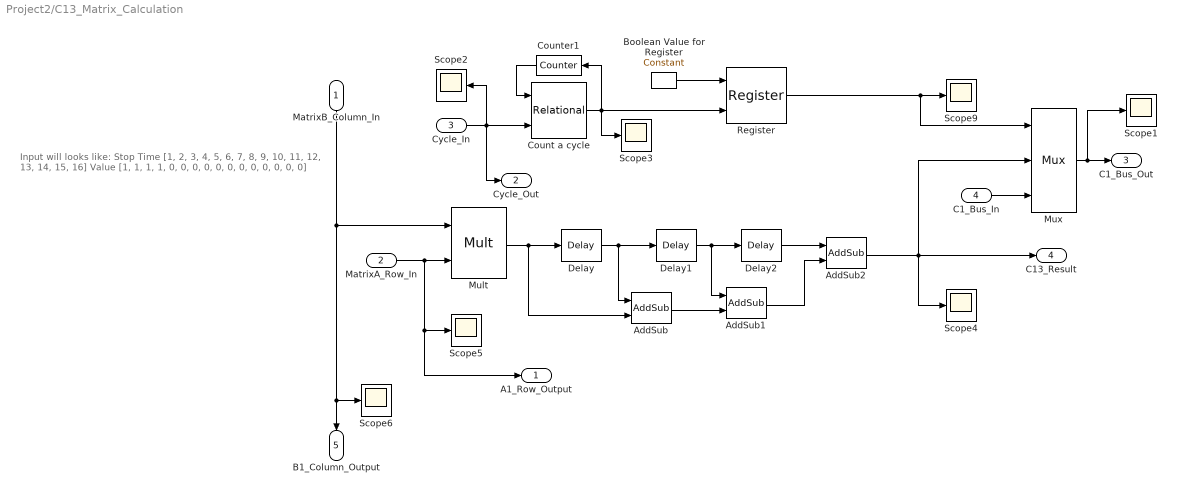
== system Project2/C13_Matrix_Calculation ==
  note: Input will looks like:
      | Stop Time [1, 2, 3, 4, 5, 6, 7, 8, 9, 10, 11, 12, 13, 14, 15, 16]
      | Value [1, 1, 1, 1, 0, 0, 0, 0, 0, 0, 0, 0, 0, 0, 0, 0]
  MatrixB_Column_In : Inport
  MatrixA_Row_In : Inport  Port=2
  Cycle_In : Inport  Port=3
  C1_Bus_In : Inport  Port=4
  AddSub : hdlBasic/AddSub  mode=Addition  use_carryin=off  use_carryout=off  en=off  latency=0  precision=Full  arith_type=Unsigned  n_bits=16  bin_pt=14  quantization=Truncate  overflow=Wrap  use_behavioral_HDL=off  hw_selection=Fabric  pipelined=off  XmcBlockStatus=1  maskContainerNames=tabcontainer1  block_type=addsub  block_config=sysgen:Addsub_config
  AddSub1 : hdlBasic/AddSub  mode=Addition  use_carryin=off  use_carryout=off  en=off  latency=0  precision=Full  arith_type=Unsigned  n_bits=16  bin_pt=14  quantization=Truncate  overflow=Wrap  use_behavioral_HDL=off  hw_selection=Fabric  pipelined=off  XmcBlockStatus=1  maskContainerNames=tabcontainer1  block_type=addsub  block_config=sysgen:Addsub_config
  AddSub2 : hdlBasic/AddSub  mode=Addition  use_carryin=off  use_carryout=off  en=off  latency=0  precision=Full  arith_type=Unsigned  n_bits=16  bin_pt=14  quantization=Truncate  overflow=Wrap  use_behavioral_HDL=off  hw_selection=Fabric  pipelined=off  XmcBlockStatus=1  maskContainerNames=tabcontainer1  block_type=addsub  block_config=sysgen:Addsub_config
  Boolean Value for Register : hdlBasic/Constant  const=1.0  gui_display_data_type=Boolean  arith_type=Boolean  n_bits=16  bin_pt=14  preci_type=Single  exp_width=8  frac_width=24  explicit_period=off  period=1  XmcBlockStatus=1  maskContainerNames=tabcontainer1  block_type=constant  block_config=sysgen:Constant_config
  Count a cycle : hdlBasic/Relational  mode=a=b  op_type=Bool  en=off  latency=1  XmcBlockStatus=1  maskContainerNames=tabcontainer1  block_type=relational  block_config=sysgen:Relational_config
  Counter1 : hdlBasic/Counter  cnt_type=Free running  cnt_to=8  operation=Up  start_count=0  cnt_by_val=1  arith_type=Unsigned  n_bits=6  bin_pt=0  load_pin=off  rst=on  en=off  explicit_period=Explicit  period=1  use_behavioral_HDL=off  implementation=Fabric  XmcBlockStatus=1  maskContainerNames=group1  block_type=counter  block_config=sysgen:Counter_config
  Delay : hdlBasic/Delay  rst=off  en=off  latency=1  reg_retiming=off  XmcBlockStatus=1  maskContainerNames=group1  block_type=delay  block_config=sysgen:Delay_config
  Delay1 : hdlBasic/Delay  rst=off  en=off  latency=1  reg_retiming=off  XmcBlockStatus=1  maskContainerNames=group1  block_type=delay  block_config=sysgen:Delay_config
  Delay2 : hdlBasic/Delay  rst=off  en=off  latency=1  reg_retiming=off  XmcBlockStatus=1  maskContainerNames=group1  block_type=delay  block_config=sysgen:Delay_config
  Mult : hdlBasic/Mult  precision=Full  arith_type="Signed  (2's comp)"  n_bits=16  bin_pt=14  quantization=Truncate  overflow=Wrap  en=off  latency=3  use_behavioral_HDL=off  opt=Speed  use_embedded=on  optimum_pipeline=off  pipeline=on  use_rpm=on  placement_style=Triangular  XmcBlockStatus=1  maskContainerNames=group1  block_type=mult  block_config=sysgen:Mult_config
  Mux : hdlBasic/Mux  inputs=2  en=off  latency=1  precision=Full  arith_type=Unsigned  n_bits=16  bin_pt=14  quantization=Truncate  overflow=Wrap  XmcBlockStatus=1  maskContainerNames=tabcontainer1  block_type=mux  block_config=sysgen:Mux_config
  Register : hdlBasic/Register  init=0  rst=on  en=off  XmcBlockStatus=1  maskContainerNames=tabcontainer1  block_type=register  block_config=sysgen:Register_config
  Scope{1..6,9} (7 alike) : Scope
  A1_Row_Output : Outport
  Cycle_Out : Outport  Port=2
  C1_Bus_Out : Outport  Port=3
  C13_Result : Outport  Port=4
  B1_Column_Output : Outport  Port=5
  wires:
  MatrixB_Column_In/1 -> Scope6/1, B1_Column_Output/1, Mult/1
  MatrixA_Row_In/1 -> Scope5/1, A1_Row_Output/1, Mult/2
  Mult/1 -> Delay/1, AddSub/2
  AddSub/1 -> AddSub1/2
  Delay/1 -> AddSub/1, Delay1/1
  Delay1/1 -> Delay2/1, AddSub1/1
  AddSub1/1 -> AddSub2/2
  Delay2/1 -> AddSub2/1
  AddSub2/1 -> Scope4/1, Mux/2, C13_Result/1
  Count a cycle/1 -> Register/2, Counter1/1, Scope3/1
  Counter1/1 -> Count a cycle/1
  Mux/1 -> Scope1/1, C1_Bus_Out/1
  Register/1 -> Mux/1, Scope9/1
  Boolean Value for Register/1 -> Register/1
  C1_Bus_In/1 -> Mux/3
  Cycle_In/1 -> Cycle_Out/1, Count a cycle/2, Scope2/1

== system Project2/C14_Matrix_Calculation ==
  note: Input will looks like:
      | Stop Time [1, 2, 3, 4, 5, 6, 7, 8, 9, 10, 11, 12, 13, 14, 15, 16]
      | Value [1, 1, 1, 1, 0, 0, 0, 0, 0, 0, 0, 0, 0, 0, 0, 0]
  MatrixB_Column_In : Inport
  MatrixA_Row_In : Inport  Port=2
  Cycle_In : Inport  Port=3
  C1_Bus_In : Inport  Port=4
  AddSub : hdlBasic/AddSub  mode=Addition  use_carryin=off  use_carryout=off  en=off  latency=0  precision=Full  arith_type=Unsigned  n_bits=16  bin_pt=14  quantization=Truncate  overflow=Wrap  use_behavioral_HDL=off  hw_selection=Fabric  pipelined=off  XmcBlockStatus=1  maskContainerNames=tabcontainer1  block_type=addsub  block_config=sysgen:Addsub_config
  AddSub1 : hdlBasic/AddSub  mode=Addition  use_carryin=off  use_carryout=off  en=off  latency=0  precision=Full  arith_type=Unsigned  n_bits=16  bin_pt=14  quantization=Truncate  overflow=Wrap  use_behavioral_HDL=off  hw_selection=Fabric  pipelined=off  XmcBlockStatus=1  maskContainerNames=tabcontainer1  block_type=addsub  block_config=sysgen:Addsub_config
  AddSub2 : hdlBasic/AddSub  mode=Addition  use_carryin=off  use_carryout=off  en=off  latency=0  precision=Full  arith_type=Unsigned  n_bits=16  bin_pt=14  quantization=Truncate  overflow=Wrap  use_behavioral_HDL=off  hw_selection=Fabric  pipelined=off  XmcBlockStatus=1  maskContainerNames=tabcontainer1  block_type=addsub  block_config=sysgen:Addsub_config
  Boolean Value for Register : hdlBasic/Constant  const=1.0  gui_display_data_type=Boolean  arith_type=Boolean  n_bits=16  bin_pt=14  preci_type=Single  exp_width=8  frac_width=24  explicit_period=off  period=1  XmcBlockStatus=1  maskContainerNames=tabcontainer1  block_type=constant  block_config=sysgen:Constant_config
  Count a cycle : hdlBasic/Relational  mode=a=b  op_type=Bool  en=off  latency=1  XmcBlockStatus=1  maskContainerNames=tabcontainer1  block_type=relational  block_config=sysgen:Relational_config
  Counter1 : hdlBasic/Counter  cnt_type=Free running  cnt_to=8  operation=Up  start_count=0  cnt_by_val=1  arith_type=Unsigned  n_bits=6  bin_pt=0  load_pin=off  rst=on  en=off  explicit_period=Explicit  period=1  use_behavioral_HDL=off  implementation=Fabric  XmcBlockStatus=1  maskContainerNames=group1  block_type=counter  block_config=sysgen:Counter_config
  Delay : hdlBasic/Delay  rst=off  en=off  latency=1  reg_retiming=off  XmcBlockStatus=1  maskContainerNames=group1  block_type=delay  block_config=sysgen:Delay_config
  Delay1 : hdlBasic/Delay  rst=off  en=off  latency=1  reg_retiming=off  XmcBlockStatus=1  maskContainerNames=group1  block_type=delay  block_config=sysgen:Delay_config
  Delay2 : hdlBasic/Delay  rst=off  en=off  latency=1  reg_retiming=off  XmcBlockStatus=1  maskContainerNames=group1  block_type=delay  block_config=sysgen:Delay_config
  Mult : hdlBasic/Mult  precision=Full  arith_type="Signed  (2's comp)"  n_bits=16  bin_pt=14  quantization=Truncate  overflow=Wrap  en=off  latency=3  use_behavioral_HDL=off  opt=Speed  use_embedded=on  optimum_pipeline=off  pipeline=on  use_rpm=on  placement_style=Triangular  XmcBlockStatus=1  maskContainerNames=group1  block_type=mult  block_config=sysgen:Mult_config
  Mux : hdlBasic/Mux  inputs=2  en=off  latency=1  precision=Full  arith_type=Unsigned  n_bits=16  bin_pt=14  quantization=Truncate  overflow=Wrap  XmcBlockStatus=1  maskContainerNames=tabcontainer1  block_type=mux  block_config=sysgen:Mux_config
  Register : hdlBasic/Register  init=0  rst=on  en=off  XmcBlockStatus=1  maskContainerNames=tabcontainer1  block_type=register  block_config=sysgen:Register_config
  Scope{1..6,9} (7 alike) : Scope
  C1_Bus_Out : Outport
  C14 Result : Outport  Port=2
  B1_Column_Output : Outport  Port=3
  wires:
  MatrixB_Column_In/1 -> Scope4/1, B1_Column_Output/1, Mult/1
  Mult/1 -> Delay/1, AddSub/2
  AddSub/1 -> AddSub1/2
  Delay/1 -> AddSub/1, Delay1/1
  Delay1/1 -> Delay2/1, AddSub1/1
  AddSub1/1 -> AddSub2/2
  Delay2/1 -> AddSub2/1
  AddSub2/1 -> C14 Result/1, Scope5/1, Mux/2
  Boolean Value for Register/1 -> Register/1
  Register/1 -> Mux/1, Scope9/1
  C1_Bus_In/1 -> Mux/3
  Count a cycle/1 -> Register/2, Counter1/1, Scope3/1
  Mux/1 -> Scope1/1, C1_Bus_Out/1
  Counter1/1 -> Count a cycle/1
  Cycle_In/1 -> Count a cycle/2, Scope2/1
  MatrixA_Row_In/1 -> Scope6/1, Mult/2

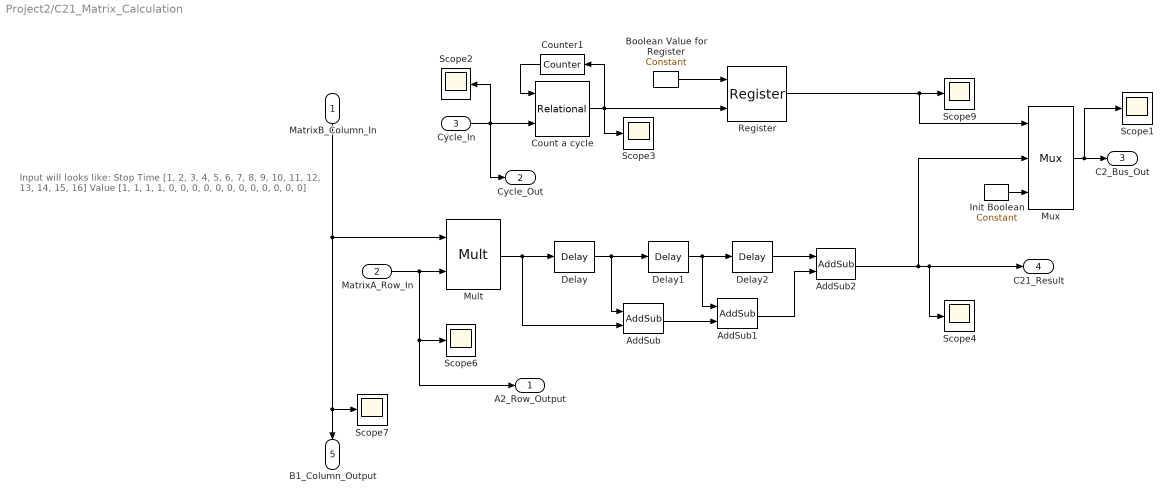
== system Project2/C21_Matrix_Calculation ==
  note: Input will looks like:
      | Stop Time [1, 2, 3, 4, 5, 6, 7, 8, 9, 10, 11, 12, 13, 14, 15, 16]
      | Value [1, 1, 1, 1, 0, 0, 0, 0, 0, 0, 0, 0, 0, 0, 0, 0]
  MatrixB_Column_In : Inport
  MatrixA_Row_In : Inport  Port=2
  Cycle_In : Inport  Port=3
  AddSub : hdlBasic/AddSub  mode=Addition  use_carryin=off  use_carryout=off  en=off  latency=0  precision=Full  arith_type=Unsigned  n_bits=16  bin_pt=14  quantization=Truncate  overflow=Wrap  use_behavioral_HDL=off  hw_selection=Fabric  pipelined=off  XmcBlockStatus=1  maskContainerNames=tabcontainer1  block_type=addsub  block_config=sysgen:Addsub_config
  AddSub1 : hdlBasic/AddSub  mode=Addition  use_carryin=off  use_carryout=off  en=off  latency=0  precision=Full  arith_type=Unsigned  n_bits=16  bin_pt=14  quantization=Truncate  overflow=Wrap  use_behavioral_HDL=off  hw_selection=Fabric  pipelined=off  XmcBlockStatus=1  maskContainerNames=tabcontainer1  block_type=addsub  block_config=sysgen:Addsub_config
  AddSub2 : hdlBasic/AddSub  mode=Addition  use_carryin=off  use_carryout=off  en=off  latency=0  precision=Full  arith_type=Unsigned  n_bits=16  bin_pt=14  quantization=Truncate  overflow=Wrap  use_behavioral_HDL=off  hw_selection=Fabric  pipelined=off  XmcBlockStatus=1  maskContainerNames=tabcontainer1  block_type=addsub  block_config=sysgen:Addsub_config
  Boolean Value for Register : hdlBasic/Constant  const=1.0  gui_display_data_type=Boolean  arith_type=Boolean  n_bits=16  bin_pt=14  preci_type=Single  exp_width=8  frac_width=24  explicit_period=off  period=1  XmcBlockStatus=1  maskContainerNames=tabcontainer1  block_type=constant  block_config=sysgen:Constant_config
  Count a cycle : hdlBasic/Relational  mode=a=b  op_type=Bool  en=off  latency=1  XmcBlockStatus=1  maskContainerNames=tabcontainer1  block_type=relational  block_config=sysgen:Relational_config
  Counter1 : hdlBasic/Counter  cnt_type=Free running  cnt_to=8  operation=Up  start_count=0  cnt_by_val=1  arith_type=Unsigned  n_bits=6  bin_pt=0  load_pin=off  rst=on  en=off  explicit_period=Explicit  period=1  use_behavioral_HDL=off  implementation=Fabric  XmcBlockStatus=1  maskContainerNames=group1  block_type=counter  block_config=sysgen:Counter_config
  Delay : hdlBasic/Delay  rst=off  en=off  latency=1  reg_retiming=off  XmcBlockStatus=1  maskContainerNames=group1  block_type=delay  block_config=sysgen:Delay_config
  Delay1 : hdlBasic/Delay  rst=off  en=off  latency=1  reg_retiming=off  XmcBlockStatus=1  maskContainerNames=group1  block_type=delay  block_config=sysgen:Delay_config
  Delay2 : hdlBasic/Delay  rst=off  en=off  latency=1  reg_retiming=off  XmcBlockStatus=1  maskContainerNames=group1  block_type=delay  block_config=sysgen:Delay_config
  Init Boolean : hdlBasic/Constant  const=0  gui_display_data_type=Fixed-point  arith_type=Signed (2's comp)  n_bits=16  bin_pt=14  preci_type=Single  exp_width=8  frac_width=24  explicit_period=off  period=1  XmcBlockStatus=1  maskContainerNames=tabcontainer1  block_type=constant  block_config=sysgen:Constant_config
  Mult : hdlBasic/Mult  precision=Full  arith_type="Signed  (2's comp)"  n_bits=16  bin_pt=14  quantization=Truncate  overflow=Wrap  en=off  latency=3  use_behavioral_HDL=off  opt=Speed  use_embedded=on  optimum_pipeline=off  pipeline=on  use_rpm=on  placement_style=Triangular  XmcBlockStatus=1  maskContainerNames=group1  block_type=mult  block_config=sysgen:Mult_config
  Mux : hdlBasic/Mux  inputs=2  en=off  latency=1  precision=Full  arith_type=Unsigned  n_bits=16  bin_pt=14  quantization=Truncate  overflow=Wrap  XmcBlockStatus=1  maskContainerNames=tabcontainer1  block_type=mux  block_config=sysgen:Mux_config
  Register : hdlBasic/Register  init=0  rst=on  en=off  XmcBlockStatus=1  maskContainerNames=tabcontainer1  block_type=register  block_config=sysgen:Register_config
  Scope{1..4,6..7,9} (7 alike) : Scope
  A2_Row_Output : Outport
  Cycle_Out : Outport  Port=2
  C2_Bus_Out : Outport  Port=3
  C21_Result : Outport  Port=4
  B1_Column_Output : Outport  Port=5
  wires:
  Mult/1 -> Delay/1, AddSub/2
  AddSub/1 -> AddSub1/2
  Delay/1 -> AddSub/1, Delay1/1
  Delay1/1 -> Delay2/1, AddSub1/1
  AddSub1/1 -> AddSub2/2
  Delay2/1 -> AddSub2/1
  AddSub2/1 -> Scope4/1, C21_Result/1, Mux/2
  MatrixB_Column_In/1 -> Scope7/1, B1_Column_Output/1, Mult/1
  MatrixA_Row_In/1 -> Scope6/1, A2_Row_Output/1, Mult/2
  Counter1/1 -> Count a cycle/1
  Count a cycle/1 -> Register/2, Counter1/1, Scope3/1
  Boolean Value for Register/1 -> Register/1
  Register/1 -> Mux/1, Scope9/1
  Cycle_In/1 -> Cycle_Out/1, Count a cycle/2, Scope2/1
  Init Boolean/1 -> Mux/3
  Mux/1 -> Scope1/1, C2_Bus_Out/1

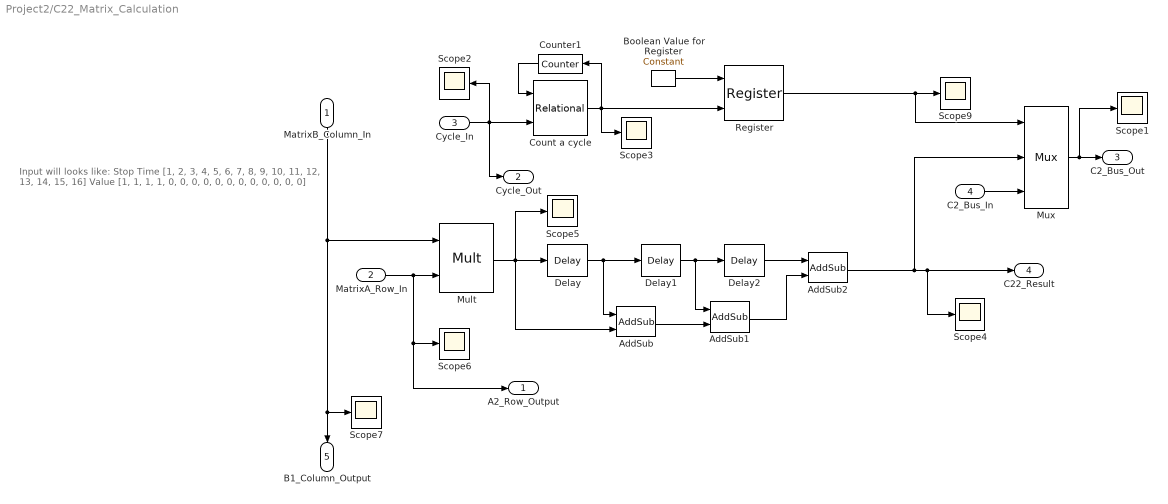
== system Project2/C22_Matrix_Calculation ==
  note: Input will looks like:
      | Stop Time [1, 2, 3, 4, 5, 6, 7, 8, 9, 10, 11, 12, 13, 14, 15, 16]
      | Value [1, 1, 1, 1, 0, 0, 0, 0, 0, 0, 0, 0, 0, 0, 0, 0]
  MatrixB_Column_In : Inport
  MatrixA_Row_In : Inport  Port=2
  Cycle_In : Inport  Port=3
  C2_Bus_In : Inport  Port=4
  AddSub : hdlBasic/AddSub  mode=Addition  use_carryin=off  use_carryout=off  en=off  latency=0  precision=Full  arith_type=Unsigned  n_bits=16  bin_pt=14  quantization=Truncate  overflow=Wrap  use_behavioral_HDL=off  hw_selection=Fabric  pipelined=off  XmcBlockStatus=1  maskContainerNames=tabcontainer1  block_type=addsub  block_config=sysgen:Addsub_config
  AddSub1 : hdlBasic/AddSub  mode=Addition  use_carryin=off  use_carryout=off  en=off  latency=0  precision=Full  arith_type=Unsigned  n_bits=16  bin_pt=14  quantization=Truncate  overflow=Wrap  use_behavioral_HDL=off  hw_selection=Fabric  pipelined=off  XmcBlockStatus=1  maskContainerNames=tabcontainer1  block_type=addsub  block_config=sysgen:Addsub_config
  AddSub2 : hdlBasic/AddSub  mode=Addition  use_carryin=off  use_carryout=off  en=off  latency=0  precision=Full  arith_type=Unsigned  n_bits=16  bin_pt=14  quantization=Truncate  overflow=Wrap  use_behavioral_HDL=off  hw_selection=Fabric  pipelined=off  XmcBlockStatus=1  maskContainerNames=tabcontainer1  block_type=addsub  block_config=sysgen:Addsub_config
  Boolean Value for Register : hdlBasic/Constant  const=1.0  gui_display_data_type=Boolean  arith_type=Boolean  n_bits=16  bin_pt=14  preci_type=Single  exp_width=8  frac_width=24  explicit_period=off  period=1  XmcBlockStatus=1  maskContainerNames=tabcontainer1  block_type=constant  block_config=sysgen:Constant_config
  Count a cycle : hdlBasic/Relational  mode=a=b  op_type=Bool  en=off  latency=1  XmcBlockStatus=1  maskContainerNames=tabcontainer1  block_type=relational  block_config=sysgen:Relational_config
  Counter1 : hdlBasic/Counter  cnt_type=Free running  cnt_to=8  operation=Up  start_count=0  cnt_by_val=1  arith_type=Unsigned  n_bits=6  bin_pt=0  load_pin=off  rst=on  en=off  explicit_period=Explicit  period=1  use_behavioral_HDL=off  implementation=Fabric  XmcBlockStatus=1  maskContainerNames=group1  block_type=counter  block_config=sysgen:Counter_config
  Delay : hdlBasic/Delay  rst=off  en=off  latency=1  reg_retiming=off  XmcBlockStatus=1  maskContainerNames=group1  block_type=delay  block_config=sysgen:Delay_config
  Delay1 : hdlBasic/Delay  rst=off  en=off  latency=1  reg_retiming=off  XmcBlockStatus=1  maskContainerNames=group1  block_type=delay  block_config=sysgen:Delay_config
  Delay2 : hdlBasic/Delay  rst=off  en=off  latency=1  reg_retiming=off  XmcBlockStatus=1  maskContainerNames=group1  block_type=delay  block_config=sysgen:Delay_config
  Mult : hdlBasic/Mult  precision=Full  arith_type="Signed  (2's comp)"  n_bits=16  bin_pt=14  quantization=Truncate  overflow=Wrap  en=off  latency=3  use_behavioral_HDL=off  opt=Speed  use_embedded=on  optimum_pipeline=off  pipeline=on  use_rpm=on  placement_style=Triangular  XmcBlockStatus=1  maskContainerNames=group1  block_type=mult  block_config=sysgen:Mult_config
  Mux : hdlBasic/Mux  inputs=2  en=off  latency=1  precision=Full  arith_type=Unsigned  n_bits=16  bin_pt=14  quantization=Truncate  overflow=Wrap  XmcBlockStatus=1  maskContainerNames=tabcontainer1  block_type=mux  block_config=sysgen:Mux_config
  Register : hdlBasic/Register  init=0  rst=on  en=off  XmcBlockStatus=1  maskContainerNames=tabcontainer1  block_type=register  block_config=sysgen:Register_config
  Scope{1..7,9} (8 alike) : Scope
  A2_Row_Output : Outport
  Cycle_Out : Outport  Port=2
  C2_Bus_Out : Outport  Port=3
  C22_Result : Outport  Port=4
  B1_Column_Output : Outport  Port=5
  wires:
  MatrixA_Row_In/1 -> Scope6/1, A2_Row_Output/1, Mult/2
  AddSub/1 -> AddSub1/2
  AddSub1/1 -> AddSub2/2
  Delay2/1 -> AddSub2/1
  Mult/1 -> Scope5/1, Delay/1, AddSub/2
  Delay1/1 -> Delay2/1, AddSub1/1
  Delay/1 -> AddSub/1, Delay1/1
  C2_Bus_In/1 -> Mux/3
  Mux/1 -> Scope1/1, C2_Bus_Out/1
  Register/1 -> Mux/1, Scope9/1
  Boolean Value for Register/1 -> Register/1
  Count a cycle/1 -> Register/2, Counter1/1, Scope3/1
  Counter1/1 -> Count a cycle/1
  AddSub2/1 -> Mux/2, Scope4/1, C22_Result/1
  MatrixB_Column_In/1 -> Mult/1, Scope7/1, B1_Column_Output/1
  Cycle_In/1 -> Cycle_Out/1, Count a cycle/2, Scope2/1
